simulink model "Single_Phase_Fully_Controlled_Converter"  (R2020b)
settings: Solver=VariableStepAuto  StartTime=0.0  StopTime=1  RelTol=1e-3
libraries: powerlib x10, powerlib_meascontrol x2
settings Model: NumberOfSteps=2  Creator=adima  LastModifiedBy=adima

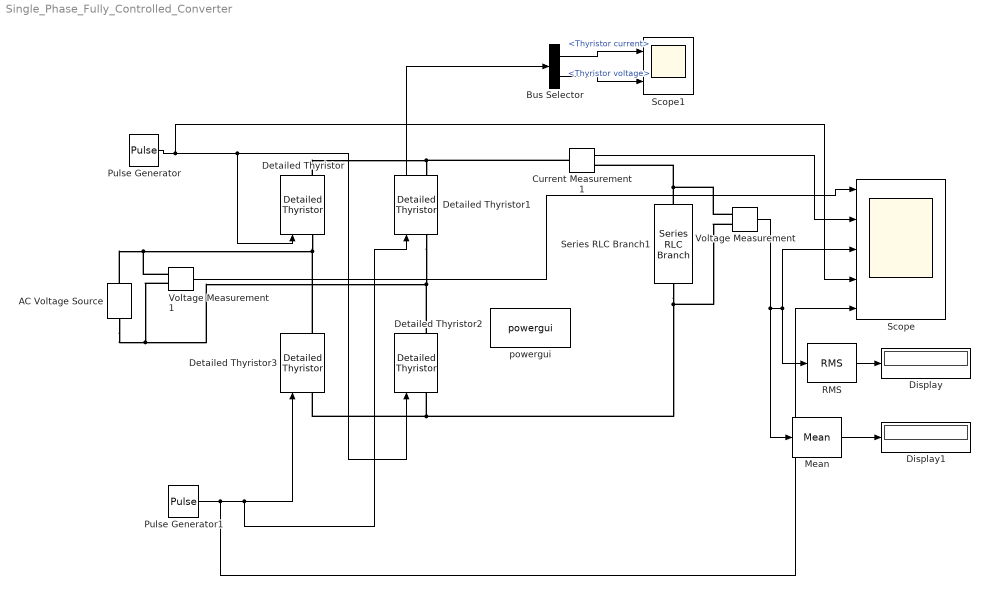
== system Single_Phase_Fully_Controlled_Converter ==
  AC Voltage Source : powerlib/Electrical Sources/AC Voltage Source  Amplitude=230  Phase=0  Frequency=50  SampleTime=0  Measurements=None  BusType=swing  Pref=10e3  Qref=0  Qmin=-inf  Qmax=+inf
  Bus Selector : BusSelector  OutputSignals=Thyristor current,Thyristor voltage
  Current Measurement1 : powerlib/Measurements/Current Measurement  PhasorSimulation=off  OutputType=Complex  PSBequivalent=0
  Detailed Thyristor{,1..3} (4 alike) : powerlib/Power Electronics/Detailed Thyristor  Ron=0.001  Lon=1e-3  Vf=0.8  IL=0.1  Tq=100e-6  IC=0  Rs=500  Cs=250e-9  Measurements=on
      settings: SourceProductBaseCode=PS
  Display : Display
  Display1 : Display
  Mean : powerlib_meascontrol/Measurements/Mean  Freq=50  Vinit=0  Ts=0
  Pulse Generator : DiscretePulseGenerator  PulseType=Time based  Period=1/50  PulseWidth=5  PhaseDelay=30*((20e-3)/360)
  Pulse Generator1 : DiscretePulseGenerator  PulseType=Time based  Period=1/50  PulseWidth=5  PhaseDelay=210*((20e-3)/360)
  RMS : powerlib_meascontrol/Measurements/RMS  TrueRMS=on  Freq=50  RMSInit=120  Ts=0
  Scope : Scope  NumInputPorts=5
  Scope1 : Scope  NumInputPorts=2
  Series RLC Branch1 : powerlib/Elements/Series RLC Branch  LConnTagsString=__new0  RConnTagsString=__new0  BranchType=RL  Resistance=10  Inductance=10e-3  SetiL0=off  InitialCurrent=0  Capacitance=1e-6  Setx0=off  InitialVoltage=0  Measurements=None
  Voltage Measurement : powerlib/Measurements/Voltage Measurement  PhasorSimulation=off  OutputType=Complex  PSBequivalent=0
  Voltage Measurement1 : powerlib/Measurements/Voltage Measurement  PhasorSimulation=off  OutputType=Complex  PSBequivalent=0
  powergui : powerlib/powergui  Priority=1  SimulationMode=Discrete  SampleTime=5e-6  frequency=60  Iterations=50  frequencyindice=50  Pbase=100e6  ErrMax=1e-4  UnitsV=kV  UnitsW=MW  buscounter=0  FunctionMessages=off  echomessages=off  EnableUseOfTLC=off  CurrentSourceSwitches=off  DisableSnubberDevices=off  DisableRonSwitches=off  DisableVfSwitches=off  DisplayEquations=off  AutomaticDiscreteSolvers=off  SolverType=Tustin/Backward Euler (TBE)  Interpol=off  ExternalGateDelay=off  methode=off  Ts=100  x0status=blocks  SPID=on  SwTol=0  HookPort=off  NonlinearTolerance=1e-4  nMaxIteration=100  ContinueOnMaxIteration=off  RestoreLinks=warning  ResistiveCurrentMeasurement=off  Frange=[0:2:500]  Ylog=off  Xlog=on  ShowGrid=off  save=off  variable=ZData  structure=0  ZoomFFT=off  StartTime=0.0  cycles=1  DisplayStyle=1  fundamental=60  FreqAxis=off  MaxFrequency=1000  frequencyindicesteady=1  RmsSteady=1  display=off
  wires:
  Pulse Generator1/1 -> Scope/5, Detailed Thyristor3/1, Detailed Thyristor1/1
  Voltage Measurement1/1 -> Scope/1
  Voltage Measurement/1 -> Mean/1, RMS/1, Scope/3
  Current Measurement1/1 -> Scope/2
  RMS/1 -> Display/1
  Mean/1 -> Display1/1
  Pulse Generator/1 -> Scope/4, Detailed Thyristor2/1, Detailed Thyristor/1
  Detailed Thyristor1/1 -> Bus Selector/1
  Bus Selector/1 -> Scope1/1  "<Thyristor current>"
  Bus Selector/2 -> Scope1/2  "<Thyristor voltage>"
  connections:
  Detailed Thyristor/LConn1 -- Detailed Thyristor3/RConn1 -- Voltage Measurement1/LConn1 -- AC Voltage Source/RConn1
  Detailed Thyristor1/LConn1 -- Detailed Thyristor2/RConn1 -- Voltage Measurement1/LConn2 -- AC Voltage Source/LConn1
  Voltage Measurement/LConn2 -- Detailed Thyristor3/LConn1 -- Detailed Thyristor2/LConn1 -- Series RLC Branch1/RConn1
  Detailed Thyristor/RConn1 -- Current Measurement1/LConn1 -- Detailed Thyristor1/RConn1
  Series RLC Branch1/LConn1 -- Voltage Measurement/LConn1 -- Current Measurement1/RConn1
